simulink model "levitron_sim"  (Simulink 7.1)
settings: Solver=ode4  SolverMode=SingleTasking  StartTime=0.0  StopTime=200  FixedStep=0.01  MaxStep=.01  RelTol=1e-3  AbsTol=1e-6
libraries: levitron_lib x3
Description:
  | Bouncing Ball Model: Use of Zero Crossing Detection
  | 
  | A rubber ball is thrown into the air with a velocity of 15
  | meters per second from a height of 10 m.  The position
  | of the ball is shown in the lower plot of the scope, and
  | the velocity of the ball is shown in the upper plot.
  | 
  | This system uses a reset integrator to change the
  | direction of the ball as it comes into contact with
  | the ground, the zero crossing detection prevents the
  | ball from going below the ground.
settings Model: Creator=The MathWorks Inc.  LastModifiedBy=volgy  CovMetricSettings=d  ExtModeTrigMode=oneshot  ExtModeArmWhenConnect=off  ExtModeAutoUpdateStatusClock=off
settings DataIOCC: ExternalInput=[]  InitialState=[]  LimitDataPoints=off  SaveOutput=off  SaveTime=off
settings OptimizationCC: BooleanDataType=off  InlineInvariantSignals=on  BufferReusableBoundary=off
settings DebuggingCC: SaveWithParameterizedLinksMsg=none  SignalResolutionControl=TryResolveAllWithWarning  SolverPrmCheckMsg=none  MultiTaskDSMMsg=warning  MultiTaskCondExecSysMsg=none  SigSpecEnsureSampleTimeMsg=none  BusObjectLabelMismatch=none  StrictBusMsg=None
settings HardwareCC: TargetUnknown=on
settings RTWCC: IncludeERTFirstTime=on
settings CodeAppCC: CustomSymbolStrFcn=$F$N$M
settings GRTTargetCC: TargetFcnLib=ansi_tfl_tmw.mat

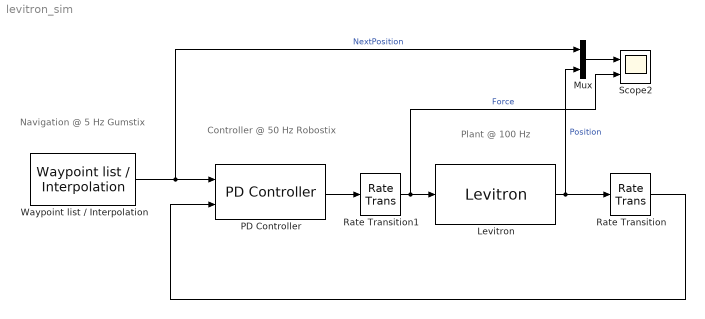
== system levitron_sim ==
  note: Controller @ 50 Hz
      | Robostix
  note: Plant @ 100 Hz
  note: Navigation @ 5 Hz
      | Gumstix
  Levitron : levitron_lib/Levitron  SystemSampleTime=-1  mass=1  gravity=-9.81  v0=15  z0=10
  Mux : Mux  Inputs=2
  PD Controller : levitron_lib/PD Controller  SystemSampleTime=-1  gain_p=6  gain_d=-5  gain=10  f_limit=100
  Rate Transition : RateTransition  OutPortSampleTime=0.02
  Rate Transition1 : RateTransition  OutPortSampleTime=0.01
  Scope2 : Scope  NumInputPorts=2
      settings: YMin=-5~0  YMax=5~50
  Waypoint list / Interpolation : levitron_lib/Waypoint list // Interpolation  SystemSampleTime=-1  sample_time=0.2  time_values=[0 20 40 60 80 100]  output_values=[10 50 30 20 40 10]
  wires:
  PD Controller/1 -> Rate Transition1/1
  Rate Transition1/1 -> Levitron/1, Scope2/2  "Force"
  Levitron/1 -> Rate Transition/1, Mux/2  "Position"
  Waypoint list / Interpolation/1 -> PD Controller/1, Mux/1  "NextPosition"
  Rate Transition/1 -> PD Controller/2
  Mux/1 -> Scope2/1
